simulink model "quad_6d_model"  (R2014a)
settings: Solver=ode45  StartTime=0.0  StopTime=10.0  RelTol=1e-3
values from neighbouring files (symbols this model uses):
  g = 9.8    [quad_mod_run.m]
  initPosLLA = [40.143237,-105.243462,1684]    [quad_mod_run.m]
  mass = 2    [quad_mod_run.m]
undefined symbols (not defined in the file or in its folder): Earth, WGS84
libraries: aerolib6dof2 x1, simulink x1, aerolibtransform2 x1
settings Model: Creator=austi_000  LastModifiedBy=austi_000

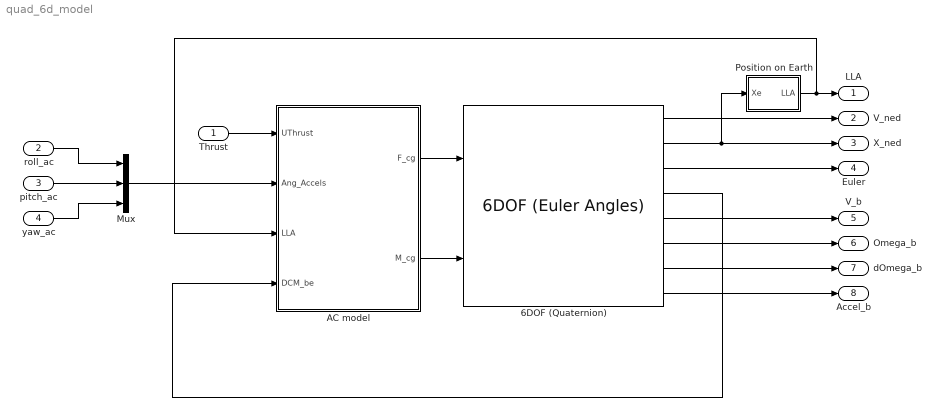
== system quad_6d_model ==
  Thrust : Inport
  roll_ac : Inport  Port=2
  pitch_ac : Inport  Port=3
  yaw_ac : Inport  Port=4
  6DOF (Quaternion) : aerolib6dof2/6DOF (Euler Angles)  units=Metric (MKS)  mtype=Fixed  rep=Quaternion  xme_0=initPosNED  Vm_0=initVb  eul_0=initEuler  pm_0=initAngRates  mass_0=mass  mass_e=0.5  mass_f=2.0  inertia=inertia  inertia_e=eye(3)  inertia_f=2*eye(3)  k_quat=1.0  vre_flag=on
  AC model : Subsystem
  Mux : Mux  Inputs=3
  Position on Earth : Subsystem  Priority=1  TreatAsAtomicUnit=on
  LLA : Outport
  V_ned : Outport  Port=2
  X_ned : Outport  Port=3
  Euler : Outport  Port=4
  V_b : Outport  Port=5
  Omega_b : Outport  Port=6
  dOmega_b : Outport  Port=7
  Accel_b : Outport  Port=8
  wires:
  AC model/1(F_cg) -> 6DOF (Quaternion)/1
  AC model/2(M_cg) -> 6DOF (Quaternion)/2
  6DOF (Quaternion)/1 -> V_ned/1
  6DOF (Quaternion)/2 -> X_ned/1, Position on Earth/1(Xe)
  6DOF (Quaternion)/3 -> Euler/1
  6DOF (Quaternion)/6 -> Omega_b/1
  6DOF (Quaternion)/7 -> dOmega_b/1
  6DOF (Quaternion)/8 -> Accel_b/1
  Position on Earth/1(LLA) -> LLA/1, AC model/3(LLA)
  6DOF (Quaternion)/5 -> V_b/1
  6DOF (Quaternion)/4 -> AC model/4(DCM_be)
  Thrust/1 -> AC model/1(UThrust)
  Mux/1 -> AC model/2(Ang_Accels)
  roll_ac/1 -> Mux/1
  pitch_ac/1 -> Mux/2
  yaw_ac/1 -> Mux/3

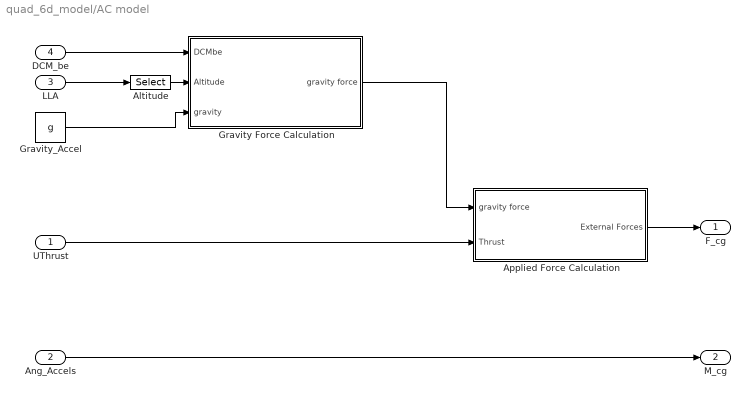
== system quad_6d_model/AC model ==
  UThrust : Inport
  Ang_Accels : Inport  Port=2
  LLA : Inport  Port=3
  DCM_be : Inport  Port=4
  Altitude : Selector  InputPortWidth=3  Indices=[3]
  Applied Force Calculation : Subsystem
  Gravity Force Calculation : Subsystem
  Gravity_Accel : Constant  Value=g
  F_cg : Outport
  M_cg : Outport  Port=2
  wires:
  Applied Force Calculation/1(External Forces) -> F_cg/1
  Gravity Force Calculation/1(gravity force) -> Applied Force Calculation/1(gravity force)
  Altitude/1 -> Gravity Force Calculation/2(Altitude)
  DCM_be/1 -> Gravity Force Calculation/1(DCMbe)
  LLA/1 -> Altitude/1
  Gravity_Accel/1 -> Gravity Force Calculation/3(gravity)
  UThrust/1 -> Applied Force Calculation/2(Thrust)
  Ang_Accels/1 -> M_cg/1

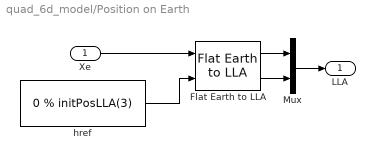
== system quad_6d_model/Position on Earth ==
  Xe : Inport
  Flat Earth to LLA : aerolibtransform2/Flat Earth to LLA  units=Metric (MKS)  ptype=Earth (WGS84)  F=1/298.257223563  R=6378137  LL0=initPosLLA(1:2)  psi=d_fn
  Mux : Mux  Inputs=2
  href : Constant  Value=0 % initPosLLA(3)
  LLA : Outport
  wires:
  Mux/1 -> LLA/1
  Xe/1 -> Flat Earth to LLA/1
  Flat Earth to LLA/1 -> Mux/1
  Flat Earth to LLA/2 -> Mux/2
  href/1 -> Flat Earth to LLA/2

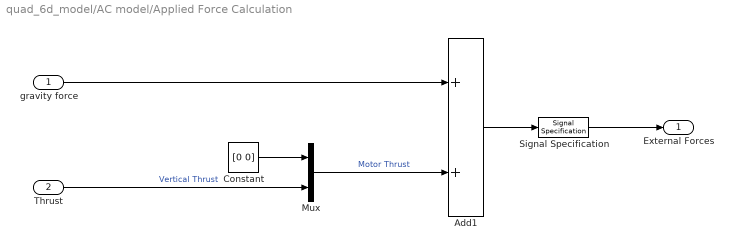
== system quad_6d_model/AC model/Applied Force Calculation ==
  gravity force : Inport
  Thrust : Inport  Port=2
  Add1 : Sum
  Constant : Constant  Value=[0 0]
  Mux : Mux  Inputs=2
  Signal Specification : SignalSpecification  Dimensions=3
  External Forces : Outport
  wires:
  Thrust/1 -> Mux/2  "Vertical Thrust"
  Constant/1 -> Mux/1
  Add1/1 -> Signal Specification/1
  Mux/1 -> Add1/2  "Motor Thrust"
  gravity force/1 -> Add1/1
  Signal Specification/1 -> External Forces/1

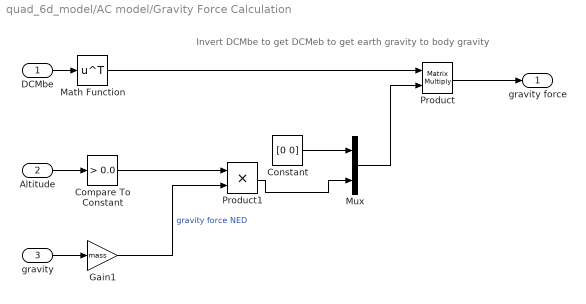
== system quad_6d_model/AC model/Gravity Force Calculation ==
  note: Invert DCMbe to get DCMeb to get earth gravity to body gravity
  DCMbe : Inport
  Altitude : Inport  Port=2
  gravity : Inport  Port=3
  Compare To Constant : simulink/Logic and Bit Operations/Compare To Constant  relop=>  const=0.0  OutDataTypeStr=boolean
  Constant : Constant  Value=[0 0]
  Gain1 : Gain  Gain=mass
  Math Function : Math  Operator=transpose  SaturateOnIntegerOverflow=on
  Mux : Mux  Inputs=2
  Product : Product  Multiplication=Matrix(*)
  Product1 : Product
  gravity force : Outport
  wires:
  gravity/1 -> Gain1/1
  Gain1/1 -> Product1/2  "gravity force NED"
  Product/1 -> gravity force/1
  Compare To Constant/1 -> Product1/1
  Altitude/1 -> Compare To Constant/1
  DCMbe/1 -> Math Function/1
  Math Function/1 -> Product/1
  Product1/1 -> Mux/2
  Constant/1 -> Mux/1
  Mux/1 -> Product/2
